simulink model "PendoloInverso"  (R2022a)
settings: Solver=VariableStepAuto  StartTime=0.0  StopTime=25.0  FixedStep=1e-3  RelTol=1e-9
values from neighbouring files (symbols this model uses):
  A = [0,    1,   0,  0 ... (first row only)    [Assignment7.m]
  B = [    0 ... (first row only)    [Assignment7.m]
  C = [1, 0, 0, 0 ... (first row only)    [Assignment7.m]
  Ce = C(1,:)    [Assignment7.m]
  f = 1    [Assignment7.m]
  g = 9.81    [Assignment7.m]
  K = place(A,-B,eigen)    [Assignment7.m]
  L = Gamma - K*Pi    [Assignment7.m]
  l = 1    [Assignment7.m]
  m = 1    [Assignment7.m]
  P = [   0, 0, 0 ... (first row only)    [Assignment7.m]
  Q = [0, -1, 0]    [Assignment7.m]
  w = 10    [Assignment7.m]
settings Model: Creator=loryb  LastModifiedBy=loryb

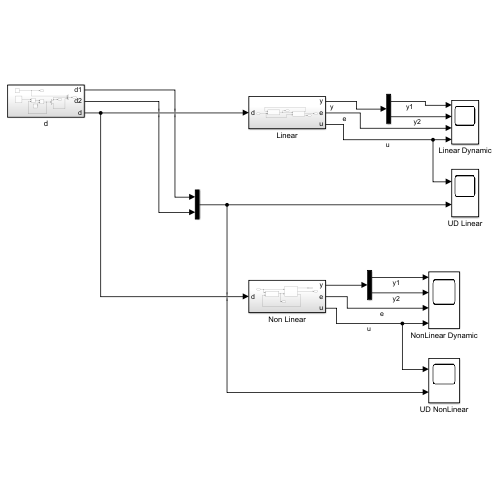
[thumbnail: Simulink's stored preview of the top-level diagram]
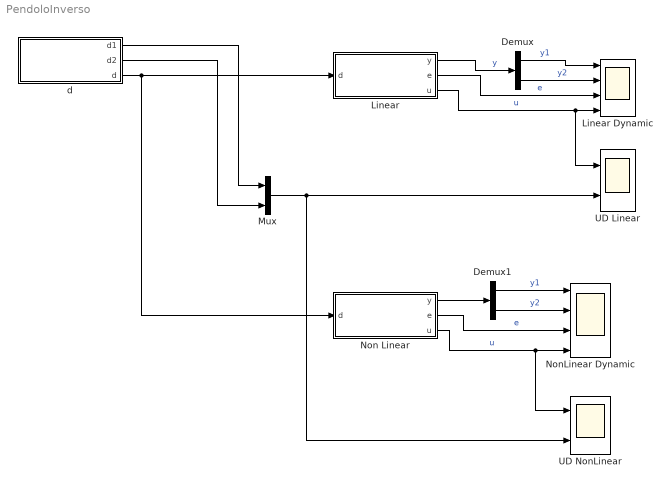
== system PendoloInverso ==
  Demux : Demux  Outputs=2
  Demux1 : Demux  Outputs=2
  Linear : Subsystem
  Linear Dynamic : Scope  NumInputPorts=4
  Mux : Mux  Inputs=2
  Non Linear : Subsystem
  NonLinear Dynamic : Scope  NumInputPorts=4
  UD Linear : Scope  NumInputPorts=2
  UD NonLinear : Scope  NumInputPorts=2
  d : Subsystem
  wires:
  d/3(d) -> Linear/1(d), Non Linear/1(d)
  Linear/1(y) -> Demux/1  "y"
  Demux/1 -> Linear Dynamic/1  "y1"
  Demux/2 -> Linear Dynamic/2  "y2"
  Linear/2(e) -> Linear Dynamic/3  "e"
  Linear/3(u) -> UD Linear/1, Linear Dynamic/4  "u"
  d/1(d1) -> Mux/1
  d/2(d2) -> Mux/2
  Mux/1 -> UD Linear/2, UD NonLinear/2
  Non Linear/1(y) -> Demux1/1
  Demux1/1 -> NonLinear Dynamic/1  "y1"
  Demux1/2 -> NonLinear Dynamic/2  "y2"
  Non Linear/2(e) -> NonLinear Dynamic/3  "e"
  Non Linear/3(u) -> UD NonLinear/1, NonLinear Dynamic/4  "u"

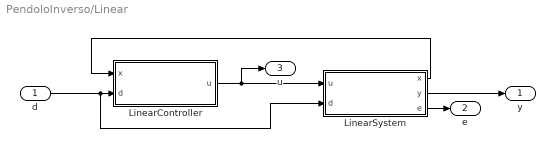
== system PendoloInverso/Linear ==
  d : Inport
  LinearController : Subsystem
  LinearSystem : Subsystem
  y : Outport
  e : Outport  Port=2
  u : Outport  Port=3
  wires:
  LinearSystem/1(x) -> LinearController/1(x)
  LinearSystem/2(y) -> y/1
  LinearSystem/3(e) -> e/1
  LinearController/1(u) -> LinearSystem/1(u), u/1
  d/1 -> LinearSystem/2(d), LinearController/2(d)

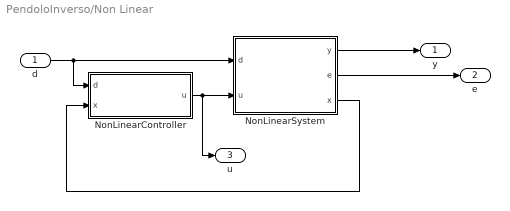
== system PendoloInverso/Non Linear ==
  d : Inport
  NonLinearController : Subsystem
  NonLinearSystem : Subsystem
  y : Outport
  e : Outport  Port=2
  u : Outport  Port=3
  wires:
  NonLinearSystem/1(y) -> y/1
  NonLinearSystem/2(e) -> e/1
  d/1 -> NonLinearController/1(d), NonLinearSystem/1(d)
  NonLinearController/1(u) -> NonLinearSystem/2(u), u/1
  NonLinearSystem/3(x) -> NonLinearController/2(x)

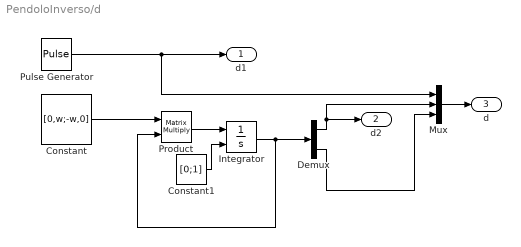
== system PendoloInverso/d ==
  Constant : Constant  Value=[0,w;-w,0]  VectorParams1D=off
  Constant1 : Constant  Value=[0;1]  VectorParams1D=off
  Demux : Demux  Outputs=2
  Integrator : Integrator  InitialConditionSource=external
  Mux : Mux  Inputs=3
  Product : Product  Multiplication=Matrix(*)
  Pulse Generator : DiscretePulseGenerator  PulseType=Time based  Amplitude=0.5  Period=50  PulseWidth=50
  d1 : Outport
  d2 : Outport  Port=2
  d : Outport  Port=3
  wires:
  Constant/1 -> Product/1
  Product/1 -> Integrator/1
  Constant1/1 -> Integrator/2
  Integrator/1 -> Demux/1, Product/2
  Demux/1 -> Mux/2, d2/1
  Demux/2 -> Mux/3
  Mux/1 -> d/1
  Pulse Generator/1 -> Mux/1, d1/1

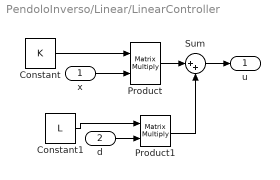
== system PendoloInverso/Linear/LinearController ==
  x : Inport
  d : Inport  Port=2
  Constant : Constant  Value=K  VectorParams1D=off
  Constant1 : Constant  Value=L  VectorParams1D=off
  Product : Product  Multiplication=Matrix(*)
  Product1 : Product  Multiplication=Matrix(*)
  Sum : Sum  Inputs=|++
  u : Outport
  wires:
  Constant/1 -> Product/1
  x/1 -> Product/2
  Constant1/1 -> Product1/1
  d/1 -> Product1/2
  Product/1 -> Sum/1
  Product1/1 -> Sum/2
  Sum/1 -> u/1

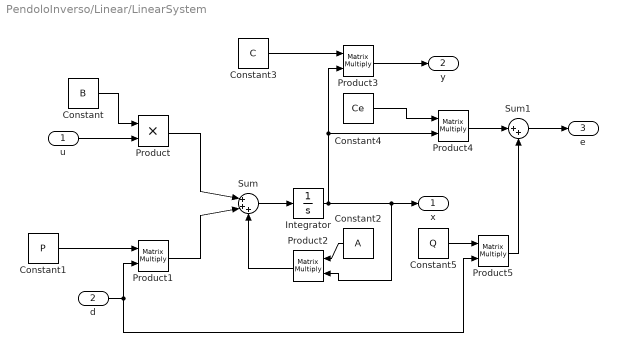
== system PendoloInverso/Linear/LinearSystem ==
  u : Inport
  d : Inport  Port=2
  Constant : Constant  Value=B  VectorParams1D=off
  Constant1 : Constant  Value=P  VectorParams1D=off
  Constant2 : Constant  Value=A  VectorParams1D=off
  Constant3 : Constant  Value=C  VectorParams1D=off
  Constant4 : Constant  Value=Ce  VectorParams1D=off
  Constant5 : Constant  Value=Q  VectorParams1D=off
  Integrator : Integrator  InitialCondition=[0;0;0;0]
  Product : Product
  Product{1..5} (5 alike) : Product  Multiplication=Matrix(*)
  Sum : Sum  Inputs=|+++
  Sum1 : Sum  Inputs=|++
  x : Outport
  y : Outport  Port=2
  e : Outport  Port=3
  wires:
  u/1 -> Product/2
  Constant/1 -> Product/1
  d/1 -> Product1/2, Product5/2
  Constant1/1 -> Product1/1
  Product/1 -> Sum/1
  Product1/1 -> Sum/2
  Sum/1 -> Integrator/1
  Product2/1 -> Sum/3
  Constant2/1 -> Product2/1
  Integrator/1 -> Product4/2, Product3/2, x/1, Product2/2
  Constant3/1 -> Product3/1
  Product3/1 -> y/1
  Constant4/1 -> Product4/1
  Product4/1 -> Sum1/1
  Constant5/1 -> Product5/1
  Product5/1 -> Sum1/2
  Sum1/1 -> e/1

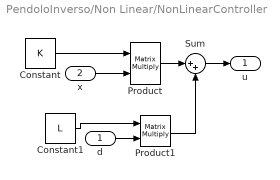
== system PendoloInverso/Non Linear/NonLinearController ==
  d : Inport
  x : Inport  Port=2
  Constant : Constant  Value=K  VectorParams1D=off
  Constant1 : Constant  Value=L  VectorParams1D=off
  Product : Product  Multiplication=Matrix(*)
  Product1 : Product  Multiplication=Matrix(*)
  Sum : Sum  Inputs=|++
  u : Outport
  wires:
  x/1 -> Product/2
  Sum/1 -> u/1
  Constant/1 -> Product/1
  d/1 -> Product1/2
  Product1/1 -> Sum/2
  Constant1/1 -> Product1/1
  Product/1 -> Sum/1

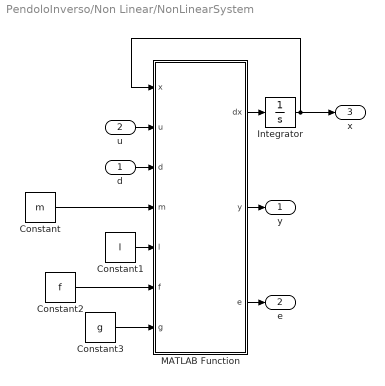
== system PendoloInverso/Non Linear/NonLinearSystem ==
  d : Inport
  u : Inport  Port=2
  Constant : Constant  Value=m
  Constant1 : Constant  Value=l
  Constant2 : Constant  Value=f
  Constant3 : Constant  Value=g
  Integrator : Integrator  InitialCondition=[0;0;0;0]
  MATLAB Function : MATLAB Function  TreatAsAtomicUnit=on
  y : Outport
  e : Outport  Port=2
  x : Outport  Port=3
  wires:
  MATLAB Function/1(dx) -> Integrator/1
  Integrator/1 -> MATLAB Function/1(x), x/1
  MATLAB Function/2(y) -> y/1
  MATLAB Function/3(e) -> e/1
  d/1 -> MATLAB Function/3(d)
  u/1 -> MATLAB Function/2(u)
  Constant/1 -> MATLAB Function/4(m)
  Constant1/1 -> MATLAB Function/5(l)
  Constant2/1 -> MATLAB Function/6(f)
  Constant3/1 -> MATLAB Function/7(g)

== matlab function PendoloInverso/Non Linear/NonLinearSystem/MATLAB Function ==
  data: x input; dx output size=4; u input; y output; d input; m input; l input; f input; g input; e output
function [dx, y, e] = fcn(x,u,d, m,l,f,g)
    dx = zeros(4,1);
    dx(1) = x(2);
    dx(2) = (-f*x(2) + u + d(1)) / m;
    dx(3) = x(4);
    dx(4) = (g*sin(x(3)) - dx(2)*cos(x(3))) / l;
    
    y = zeros(2,1);
    y(1) = x(1);
    y(2) = x(3);

    e = x(1) - d(2);
end
